simulink model "TST_DYN_MAG"  (Simulink 9.0)
settings: Solver=VariableStepAuto  StartTime=0.0  StopTime=10000  RelTol=1e-3
libraries: DYN_MAG x1, DYN_TIME x1
settings Model: Creator=Mahal  LastModifiedBy=Mahal
settings DataIOCC: SaveFormat=Dataset
settings OptimizationCC: LifeSpan=auto
settings DebuggingCC: UnderspecifiedInitializationDetection=Simplified  MergeDetectMultiDrivingBlocksExec=error  SFUnexpectedBacktrackingDiag=error  SFNoUnconditionalDefaultTransitionDiag=error  SFExecutionAtInitializationDiag=warning
settings HardwareCC: ProdBitPerPointer=64  ProdBitPerSizeT=64  ProdBitPerPtrDiffT=64  ProdLargestAtomicFloat=Float  ProdIntDivRoundTo=Zero  ProdEndianess=LittleEndian  ProdWordSize=64  ProdHWDeviceType=Intel->x86-64 (Windows64)
settings ModelReferenceCC: PropagateSignalLabelsOutOfModel=on
settings CodeAppCC: StateflowObjectComments=off
settings GRTTargetCC: TargetLangStandard=C99 (ISO)
settings ConfigComp: CovMetricSettings=dwe  CovHtmlReporting=off  CovSaveCumulativeToWorkspaceVar=off  CovSaveSingleToWorkspaceVar=off  CovExternalEMLEnable=on

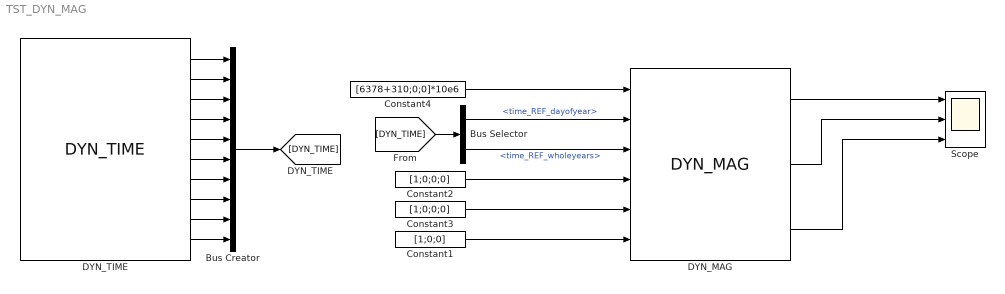
== system TST_DYN_MAG ==
  Bus Creator : BusCreator  Inputs=10
  Bus Selector : BusSelector  OutputSignals=time_REF_dayofyear,time_REF_wholeyears
  Constant1 : Constant  Value=[1;0;0]
  Constant2 : Constant  Value=[1;0;0;0]
  Constant3 : Constant  Value=[1;0;0;0]
  Constant4 : Constant  Value=[6378+310;0;0]*10e6
  DYN_MAG : DYN_MAG/DYN_MAG
  DYN_TIME : DYN_TIME/DYN_TIME
  Scope : Scope  NumInputPorts=3
  wires:
  DYN_TIME/1 -> Bus Creator/1
  DYN_TIME/2 -> Bus Creator/2
  DYN_TIME/3 -> Bus Creator/3
  DYN_TIME/4 -> Bus Creator/4
  DYN_TIME/5 -> Bus Creator/5
  DYN_TIME/6 -> Bus Creator/6
  DYN_TIME/7 -> Bus Creator/7
  DYN_TIME/8 -> Bus Creator/8
  DYN_TIME/9 -> Bus Creator/9
  DYN_TIME/10 -> Bus Creator/10
  Bus Creator/1 -> [DYN_TIME]
  DYN_MAG/1 -> Scope/1
  DYN_MAG/2 -> Scope/2
  DYN_MAG/3 -> Scope/3
  [DYN_TIME] -> Bus Selector/1
  Bus Selector/1 -> DYN_MAG/2  "<time_REF_dayofyear>"
  Bus Selector/2 -> DYN_MAG/3  "<time_REF_wholeyears>"
  Constant3/1 -> DYN_MAG/5
  Constant1/1 -> DYN_MAG/6
  Constant2/1 -> DYN_MAG/4
  Constant4/1 -> DYN_MAG/1
